simulink model "AC_SYS_SS"  (R2023b)
settings: Solver=FixedStepDiscrete  StartTime=0.0  StopTime=2  FixedStep=Ts_Power  RelTol=1e-4  EnableMultiTasking=on
PreLoadFcn:
  | HVDCMMCInterconnectionParam
StartFcn:
  | tic
StopFcn:
  | toc
values from neighbouring files (symbols this model uses):
  C_PM = 1.758e-3    (= 0.001758)    [HVDCMMCInterconnectionParam.m]
  D_R = 0.001    [HVDCMMCInterconnectionParam.m]
  D_Rs = 1e8    (= 100000000)    [HVDCMMCInterconnectionParam.m]
  Fnom = 50    [HVDCMMCInterconnectionParam.m]
  HRM = 2    [HVDCMMCInterconnectionParam.m]
  Limits_Qreg = [ 0.25, -0.25 ]    [HVDCMMCInterconnectionParam.m]
  Nb_PM = 36    [HVDCMMCInterconnectionParam.m]
  P_Ld1 = Psc/30    (= 666666666.667)    [HVDCMMCInterconnectionParam.m]
  Slope_Pref = 0.5    [HVDCMMCInterconnectionParam.m]
  Slope_Qref = 0.5    [HVDCMMCInterconnectionParam.m]
  Slope_Vdc_ref = Vnom_dc/5    (= 128000)    [HVDCMMCInterconnectionParam.m]
  Tbrk1_On = 0.1    [HVDCMMCInterconnectionParam.m]
  Tbrk2_On = 1.0    (= 1)    [HVDCMMCInterconnectionParam.m]
  Tdeblock = 1.5    [HVDCMMCInterconnectionParam.m]
  Tfault = 9999    [HVDCMMCInterconnectionParam.m]
  Ton_Converter2 = 4    [HVDCMMCInterconnectionParam.m]
  Ton_PQreg = 4    [HVDCMMCInterconnectionParam.m]
  Ton_VDCreg = 1.5    [HVDCMMCInterconnectionParam.m]
  Ts = Ts_Control    (= 4e-05)    [HVDCMMCInterconnectionParam.m]
  Ts_Power = 20e-6    (= 2e-05)    [HVDCMMCInterconnectionParam.m]
  Vb_dc = Vnom_dc    (= 640000)    [HVDCMMCInterconnectionParam.m]
  Vnom_dc = 640e3    (= 640000)    [HVDCMMCInterconnectionParam.m]
  Vnom_prim = 400e3    (= 400000)    [HVDCMMCInterconnectionParam.m]
  Vnom_sec = 333e3    (= 333000)    [HVDCMMCInterconnectionParam.m]
  w = 2*pi*Fnom    (= 314.159265359)    [HVDCMMCInterconnectionParam.m]
undefined symbols (not defined in the file or in its folder): ACSYS_T, DiscIntNeverNeededParam, Discrete, Pcc, sps_AC, spsDiodeModel
libraries: simulink x12, spsThreePhaseSeriesRLCBranchLib x7, spsGroundLib x3, spsControlledVoltageSourceLib x3, spsMultimeterLib x2, spsThreePhaseVIMeasurementLib x2, spsThreePhaseBreakerLib x1, spsThreePhaseSeriesRLCLoadLib x1, spspowerguiLib x1
(part 1 of 2)
settings Model: Creator=The MathWorks, Inc.  LastModifiedBy=rober
settings SolverCC: ConcurrentTasks=on  ZeroCrossAlgorithm=Adaptive  InsertRTBMode=Always
settings DataIOCC: SaveFormat=StructureWithTime  SaveOutput=off  SignalLogging=off  DSMLogging=off  SaveTime=off  ReturnWorkspaceOutputs=off
settings OptimizationCC: ReuseModelBlockBuffer=off  ExpressionDepthLimit=2147483647  LifeSpan=inf
settings DebuggingCC: UnderspecifiedInitializationDetection=Classic  MergeDetectMultiDrivingBlocksExec=none  SolverPrmCheckMsg=warning  FcnCallInpInsideContextMsg=warning  AllowSymbolicDim=off  StateNameClashWarn=warning  SFUnexpectedBacktrackingDiag=warning  SFNoUnconditionalDefaultTransitionDiag=warning  SFExecutionAtInitializationDiag=none  ArithmeticOperatorsInVariantConditions=warning
settings HardwareCC: ProdBitPerPointer=32  ProdBitPerSizeT=32  ProdBitPerPtrDiffT=32  ProdLargestAtomicFloat=None  ProdIntDivRoundTo=Undefined  ProdEndianess=Unspecified  ProdWordSize=32  ProdHWDeviceType=32-bit Generic
settings ModelReferenceCC: EnableRefExpFcnMdlSchedulingChecks=on  EnableParallelModelReferenceBuilds=on  ModelReferenceMinAlgLoopOccurrences=on  PropagateSignalLabelsOutOfModel=off  UseModelRefSolver=on
settings SFSimCC: SimUseLocalCustomCode=off  CustomCodeUndefinedFunction=UseInterfaceOnly
settings RTWCC: RTWUseLocalCustomCode=off
settings CodeAppCC: StateflowObjectComments=on
settings GRTTargetCC: CombineOutputUpdateFcns=off  GRTInterface=on
settings ConfigComp: CovMetricSettings=dw  CovSaveCumulativeToWorkspaceVar=on  CovSaveSingleToWorkspaceVar=on  CovExternalEMLEnable=off
settings SimscapeCC: SimscapeNormalizeSystem=off

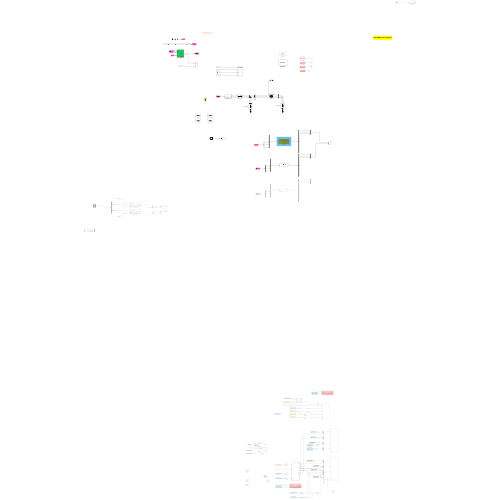
[thumbnail: Simulink's stored preview of the top-level diagram]
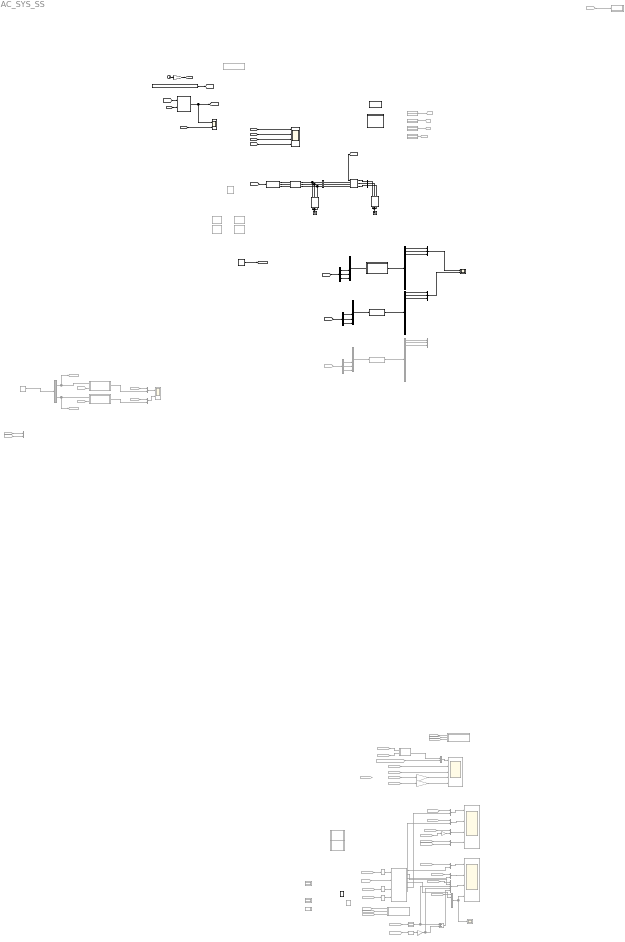
== system AC_SYS_SS ==
  note: HVDC-MMC Control System
  3ph SM1 : Subsystem  Commented=on
  3ph SM2 : Subsystem  Commented=on
  BRK_CTRL : Subsystem  Commented=on
  BRK_CTRL1 : Subsystem  Commented=on
  Brk1 : spsThreePhaseBreakerLib/Three-Phase Breaker  InitialState=open  SwitchA=on  SwitchB=on  SwitchC=on  SwitchTimes=0.1  External=on  BreakerResistance=0.0077  SnubberResistance=0.85e6  SnubberCapacitance=inf  Measurements=Breaker voltages and currents
  Brk1_RS : spsThreePhaseSeriesRLCBranchLib/Three-Phase Series RLC Branch  Commented=on  LConnTagsString=A|B|C  RConnTagsString=A|B|C  BranchType=R  Resistance=1e6  Inductance=Vnom_prim^2 / Pcc / (2*pi*Fnom)  Capacitance=1e-6  Measurements=None
  Brk1_Ron : spsThreePhaseSeriesRLCBranchLib/Three-Phase Series RLC Branch  Commented=on  LConnTagsString=A|B|C  RConnTagsString=A|B|C  BranchType=R  Resistance=0.009  Inductance=Vnom_prim^2 / Pcc / (2*pi*Fnom)  Capacitance=1e-6  Measurements=None
  Brk2_RS : spsThreePhaseSeriesRLCBranchLib/Three-Phase Series RLC Branch  Commented=on  LConnTagsString=A|B|C  RConnTagsString=A|B|C  BranchType=R  Resistance=1e6  Inductance=Vnom_prim^2 / Pcc / (2*pi*Fnom)  Capacitance=1e-6  Measurements=None
  Brk2_Ron : spsThreePhaseSeriesRLCBranchLib/Three-Phase Series RLC Branch  Commented=on  LConnTagsString=A|B|C  RConnTagsString=A|B|C  BranchType=R  Resistance=0.011  Inductance=Vnom_prim^2 / Pcc / (2*pi*Fnom)  Capacitance=1e-6  Measurements=None
  Clock : Clock
  Constant3 : Constant  Value=complex( [[ 0 Vnom_prim*sqrt(2/3); 0 0; 0 0] zeros(3,HRM-1) ])
  DQn->ABC : MATLAB Function  TreatAsAtomicUnit=on  SystemSampleTime=Ts_Power  mask{N=HRM}
      mask prompts: N "Harmonic order:"
  DSS : Subsystem  SystemSampleTime=Ts_Power  mask{A=ACSYS_T.A, B=ACSYS_T.B, C=ACSYS_T.C, D=ACSYS_T.D, InitVec=ACSYS_T.x0, dt=Ts_Power, NrBrk=3, DQSYM=off, N=HRM, Ws=w}
      mask prompts: InitVec "Initial condition:"; dt "Time step (s):"; NrBrk "Number of breakers:"; N "Harmonic number:"; Ws "Angular frequency (1/rad):"
      mask init:
      | % I = eye(size(A,1));
      | % INVR = I/(I-A*dt/2);
      | % Ad1 = INVR*(I+A*dt/2);
      | % Bd1 = INVR*B*dt/2;
      | % Cd1 = C*Ad1;
      | % Dd11 = C*INVR*B*dt/2+D;
      | % Dd12 = C*INVR*B*dt/2;
      | 
      |     I = eye(size(A,1));
      |     INVR = I/(I-A*dt/2);
      |     Ad1 = INVR*(I+A*dt/2);
      |     Bd1 = INVR*B;
      |     Cd1 = C*INVR*dt;
      |     Dd1 = Cd1*B/2 + D;
      | 
      | DQSYM = get_param(gcb,'DQSYM');
      | 
      | comp = 0;
      | 
      |     arows = size(Ad1,1)/3; %signal size
      |     acols = size(Ad1,2)/3; %signal size
      | 
      |     brows = size(Bd1,1)/3; %signal size
      |     bcols = size(Bd1,2)/3; %signal size
      | 
      |     crows = size(Cd1,1)/3; %signal size
      |     ccols = size(Cd1,2)/3; %signal size
      | 
      |     d1rows = size(Dd1,1)/3; %signal size
      |     d1cols = size(Dd1,2)/3; %signal size
      | 
      | if(strcmp(DQSYM,'on'))
      | 
      | %Calculating the PNZ matrices
      | 
      |     a = -0.5+0.866i;
      |     a2 = -0.5-0.866i;
      |     Sas = [1,a,a2;1,a2,a;1,1,1]/3;
      | 
      | 
      | 
      |     %%%%%%%%%%%%%%%%%%%%%%% Check for inconsistencies  %%%%%%%%%%%%%%%%%%%%%%%
      | 
      |     szMatA = size(A,1);
      |     iL = eye(szMatA);
      |     szMatiL = size(iL,1);
      | 
      |     if(szMatiL ~= szMatA || size(A,1) ~= size(A,2) || size(iL,1) ~= size(iL,2))
      |         error('[Int_DQN_Mat/swFeedback] check matrix A size!');
      |     end
      | 
      |     if(arows ~= brows || acols ~= ccols || crows ~= d1rows || bcols ~= d1cols)
      |         error('[Int_DQN_Mat/Initialize] the sizes of the state-space matrices!');
      |     end
      | 
      |     %%%%%%%%%%%%%%%%%%%%%%%%%%%%%%%%%%%%%%%%%%%%%%%%%%%%%%%%%%%%%%%
      | 
      | 
      |     %%%%%%%%%%%%%%%%%%%%%%% A --> Bpnz %%%%%%%%%%%%%%%%%%%%%%%
      |     Adc = complex(zeros(3*arows,3*acols));
      | 
      |     for i = 1 : arows
      |         for j = 1 : acols
      |             Adc((1:3) + (i-1)*3,(1:3) + (j-1)*3) = Sas*Ad1((1:3) + (i-1)*3,(1:3) + (j-1)*3)/Sas;
      |             %Adc((1:3) + (i-1)*3,(1:3) + (j-1)*3) = diag(diag(real(Adc((1:3) + (i-1)*3,(1:3) + (j-1)*3))));
      |             %Adc((1:3) + (i-1)*3,(1:3) + (j-1)*3) = diag(diag((Adc((1:3) + (i-1)*3,(1:3) + (j-1)*3))));
      | 
      |         end
      |     end
      |     %%%%%%%%%%%%%%%%%%%%%%%%%%%%%%%%%%%%%%%%%%%%%%%%%%%%%%%%%%%%%%%
      | 
      |     %%%%%%%%%%%%%%%%%%%%%%% B --> Bpnz %%%%%%%%%%%%%%%%%%%%%%%
      | 
      |     Bdc = complex(zeros(3*brows,3*bcols));
      | 
      |     for i = 1 : brows
      |         for j = 1 : bcols
      |             Bdc((1:3) + (i-1)*3,(1:3) + (j-1)*3) = Sas*Bd1((1:3) + (i-1)*3,(1:3) + (j-1)*3)/Sas;
      |             %Bdc((1:3) + (i-1)*3,(1:3) + (j-1)*3) = diag(diag(real(Bdc((1:3) + (i-1)*3,(1:3) + (j-1)*3))));
      |             %Bdc((1:3) + (i-1)*3,(1:3) + (j-1)*3) = diag(diag((Bdc((1:3) + (i-1)*3,(1:3) + (j-1)*3))));
      | 
      |         end
      |     end
      |     %%%%%%%%%%%%%%%%%%%%%%%%%%%%%%%%%%%%%%%%%%%%%%%%%%%%%%%%%%%%%%%
      | 
      |     %%%%%%%%%%%%%%%%%%%%%%% C --> Cpnz %%%%%%%%%%%%%%%%%%%%%%%
      | 
      |     Cdc = complex(zeros(3*crows,3*ccols));
      | 
      |     for i = 1 : crows
      |         for j = 1 : ccols
      |             Cdc((1:3) + (i-1)*3,(1:3) + (j-1)*3) = Sas*Cd1((1:3) + (i-1)*3,(1:3) + (j-1)*3)/Sas;
      |             %Cdc((1:3) + (i-1)*3,(1:3) + (j-1)*3) = diag(diag(real(Cdc((1:3) + (i-1)*3,(1:3) + (j-1)*3))));
      |             %Cdc((1:3) + (i-1)*3,(1:3) + (j-1)*3) = diag(diag((Cdc((1:3) + (i-1)*3,(1:3) + (j-1)*3))));
      |         end
      |     end
      |     %%%%%%%%%%%%%%%%%%%%%%%%%%%%%%%%%%%%%%%%%%%%%%%%%%%%%%%%%%%%%%%
      | 
      |     
      |     %%%%%%%%%%%%%%%%%%%%%%% D1 --> Cpnz %%%%%%%%%%%%%%%%%%%%%%%
      | 
      |     Ddc = complex(zeros(3*d1rows,3*d1cols));
      | 
      |     for i = 1 : d1rows
      |         for j = 1 : d1cols
      |             Ddc((1:3) + (i-1)*3,(1:3) + (j-1)*3) = Sas*Dd1((1:3) + (i-1)*3,(1:3) + (j-1)*3)/Sas;
      |             %Ddc1((1:3) + (i-1)*3,(1:3) + (j-1)*3) = diag(diag(real(Ddc1((1:3) + (i-1)*3,(1:3) + (j-1)*3))));
      |             %Ddc((1:3) + (i-1)*3,(1:3) + (j-1)*3) = diag(diag((Ddc((1:3) + (i-1)*3,(1:3) + (j-1)*3))));
      |         end
      |     end
      |     %%%%%%%%%%%%%%%%%%%%%%%%%%%%%%%%%%%%%%%%%%%%%%%%%%%%%%%%%%%%%%%
      | 
      |     Adc(abs(Adc)<2*eps) = 0;
      |     Bdc(abs(Bdc)<2*eps) = 0;
      |     Cdc(abs(Cdc)<2*eps) = 0;
      |     Ddc(abs(Ddc)<2*eps) = 0;
      | 
      |     InitVec_c = complex(zeros(brows*3,N+1));
      | 
      | 
      |     if(~isempty(InitVec))
      |         if(mod(numel(InitVec),3)~=0) 
      |             warning('[SS_DQNc_Mat] InitVec with wrong size --> needs to be a multiple of 3!'); 
      | 
      |         else
      |             for k = 1 : numel(InitVec)/3
      |                 InitVec_c((k-1)*3+1:(k-1)*3+3,1) = Sas*InitVec((k-1)*3+1:(k-1)*3+3)*exp(+1i*Ws*dt);
      |             end
      |         end
      |     end
      | 
      |     InitVec = InitVec_c;
      | 
      | 
      |     Ad1 = Adc;
      |     Bd1 = Bdc;
      |     Cd1 = Cdc;
      |     Dd1 = Ddc;
      | 
      |     comp = -1i*Ws*dt;
      | 
      | 
      | end
      | 
      |     
      |     Ad11 = Ad1(1:NrBrk,1:NrBrk);        if(isempty(Ad11)) Ad11 = zeros(3,3); end
      |     Ad12 = Ad1(1:NrBrk,NrBrk+1:end);    if(isempty(Ad12)) Ad12 = zeros(3,3); end
      |     Ad21 = Ad1(NrBrk+1:end,1:NrBrk);    if(isempty(Ad21)) Ad21 = zeros(3,3); end
      |     Ad22 = Ad1(NrBrk+1:end,NrBrk+1:end); if(isempty(Ad22)) Ad22 = zeros(3,3); end
      | 
      |     Bd11 = Bd1(1:NrBrk,1:NrBrk);        if(isempty(Bd11)) Bd11 = zeros(3,3); end
      |     Bd12 = Bd1(1:NrBrk,NrBrk+1:end);    if(isempty(Bd12)) Bd12 = zeros(3,3); end
      |     Bd21 = Bd1(NrBrk+1:end,1:NrBrk);    if(isempty(Bd21)) Bd21 = zeros(3,3); end
      |     Bd22 = Bd1(NrBrk+1:end,NrBrk+1:end); if(isempty(Bd22)) Bd22 = zeros(3,3*bcols-NrBrk); end
      | 
      |     Cd11 = Cd1(1:NrBrk,1:NrBrk);        if(isempty(Cd11)) Cd11 = zeros(3,3); end
      |     Cd12 = Cd1(1:NrBrk,NrBrk+1:end);    if(isempty(Cd12)) Cd12 = zeros(3,3); end
      |     Cd21 = Cd1(NrBrk+1:end,1:NrBrk);    if(isempty(Cd21)) Cd21 = zeros(3,3); end
      |     Cd22 = Cd1(NrBrk+1:end,NrBrk+1:end); if(isempty(Cd22)) Cd22 = zeros(3*crows-NrBrk,3*ccols); end
      | 
      |     Dd11 = Dd1(1:NrBrk,1:NrBrk);        if(isempty(Dd11)) Dd11 = zeros(3,3); end
      |     Dd12 = Dd1(1:NrBrk,NrBrk+1:end);    if(isempty(Dd12)) Dd12 = zeros(3,3); end
      |     Dd21 = Dd1(NrBrk+1:end,1:NrBrk);    if(isempty(Dd21)) Dd21 = zeros(3,3); end
      |     Dd22 = Dd1(NrBrk+1:end,NrBrk+1:end); if(isempty(Dd22)) Dd22 = zeros(3,3); end
      | 
      | 
      | 
      | 
      | InitVecS = InitVec(1:NrBrk);
      | 
      | InitVecNS = InitVec(NrBrk+1:end); if(isempty(InitVecNS)) InitVecNS = 0; end
      settings: MinAlgLoopOccurrences=on
      settings: LibrarySourceBlock=|
      | spsSynchronousMachineModel/Discrete robust/State Space Model/Discretize
      | BE or Tustin
      mask Display: disp(['{\color{red}\bf\fontsize{12}x(t) = Ad*x(t-dt)+Bd*u(t)}',newline,'{\color{gray}\bf\fontsize{12}y(t) = Cd*x(t-dt)+Dd*u(t)}'], 'texmode','on');
  Delay{,3,10..11} (4 alike) : Delay  Commented=on  DelayLength=1  SampleTime=Ts_Power
  Delay2 : Delay  DelayLength=1  SampleTime=Ts_Power
  Delay5 : Subsystem  Commented=on
  Delay6 : Subsystem  Commented=on
  Delay7 : Subsystem  Commented=on
  Delay8 : Subsystem  Commented=on
  Delay9 : Subsystem  Commented=on
  Demux : Demux  Outputs=3
  Demux1 : Demux  Outputs=3
  Demux2 : Demux  Commented=on  Outputs=3
  Demux3 : Demux  Outputs=numel(ACSYS_T.outputs)
  Demux4 : Demux  Commented=on  Outputs=2
  Demux5 : Demux  Commented=on  Outputs=numel(ACSYS_T.outputs)
  Demux6 : Demux  Outputs=numel(ACSYS_T.outputs)
  Discrete State-Space : DiscreteStateSpace  A=ACSYS_T.Adiscrete  B=ACSYS_T.Bdiscrete  C=ACSYS_T.Cdiscrete  D=ACSYS_T.Ddiscrete  InitialCondition=ACSYS_T.x0  SampleTime=Ts_Power
  Discrete State-Space1 : DiscreteStateSpace  Commented=on  A=ACSYS_T.Adiscrete  B=ACSYS_T.Bdiscrete  C=ACSYS_T.Cdiscrete  D=ACSYS_T.Ddiscrete  InitialCondition=ACSYS_T.x0  SampleTime=Ts
  From : From  Commented=on  GotoTag=Uref_Ap  TagVisibility=global
  From1 : From  Commented=on  GotoTag=Uref_An  TagVisibility=global
  From102 : From  Commented=on  GotoTag=Ap_Vin  TagVisibility=global
  From103 : From  Commented=on  GotoTag=Ap_Vbl  TagVisibility=global
  From107 : From  Commented=on  GotoTag=I_Ap_Db  TagVisibility=global
  From11 : From  Commented=on  GotoTag=Q
  From{27,44,48,113} (4 alike) : From  Commented=on  GotoTag=I_Ap_Dt  TagVisibility=global
  From118 : From  Commented=on  GotoTag=I_Ap_Db  TagVisibility=global
  From119 : From  Commented=on  GotoTag=Ap_Icap
  From{36..37,91,120} (4 alike) : From  Commented=on  GotoTag=Ap_Ipos
  From14 : From  Commented=on  GotoTag=Vsrc_ABC  TagVisibility=global
  From2 : From  Commented=on  GotoTag=P
  From25 : From  Commented=on  GotoTag=Brk1_On  TagVisibility=global
  From26 : From  Commented=on  GotoTag=UBrk1_ss
  From28 : From  Commented=on  GotoTag=U_Ap_Dt
  From29 : From  Commented=on  GotoTag=Brk2_On  TagVisibility=global
  From30 : From  Commented=on  GotoTag=IBrk2_EMT  TagVisibility=global
  From31 : From  Commented=on  GotoTag=IBrk1_EMT  TagVisibility=global
  From33 : From  Commented=on  GotoTag=UBrk2_ss
  From34 : From  Commented=on  GotoTag=Uref_Ap  TagVisibility=global
  From39 : From  Commented=on  GotoTag=U_Ap_Dt
  From4 : From  Commented=on  GotoTag=Vdc_kV
  From5 : From  Commented=on  GotoTag=V1rmsLL
  From69 : From  Commented=on  GotoTag=U_Ap_SM
  From7 : From  Commented=on  GotoTag=An_Ipos
  From85 : From  Commented=on  GotoTag=Ap_Icap
  From9 : From  Commented=on  GotoTag=An_Icap
  From90 : From  Commented=on  GotoTag=Ap_Icap
  From96 : From  Commented=on  GotoTag=Uref_Ap  TagVisibility=global
  Gain1 : Gain  Commented=on  Gain=-1
  Gain2 : Gain  Commented=on  Gain=D_Rs/(D_R+D_Rs)
  Gain4 : Gain  Commented=on  Gain=1/Vb_dc
  Gain5 : Gain  Gain=2*pi*50
  Gain7 : Gain  Commented=on  Gain=1/Vb_dc
  Goto12 : Goto  Commented=on  GotoTag=UBrk2_EMT  TagVisibility=global
  Goto13 : Goto  Commented=on  GotoTag=UBrk1_EMT  TagVisibility=global
  Ground : spsGroundLib/Ground  LConnTagsString=a
  Ground1 : spsGroundLib/Ground  LConnTagsString=a
  Ld1 : spsThreePhaseSeriesRLCLoadLib/Three-Phase Series RLC Load  Commented=on  LConnTagsString=A|B|C  Configuration=Y (grounded)  NominalVoltage=Vnom_prim  Vabc=[1e3 1e3 1e3]  Vabcp=[1e3 1e3 1e3]  NominalFrequency=Fnom  UnbalancedPower=off  ActivePower=P_Ld1  InductivePower=0  CapacitivePower=0  Pabc=[10e3 9e3 11e3]  QLabc=[100 90 110]  QCabc=[100 90 110]  Pabcp=[10e3 9e3 11e3]  QLabcp=[100 90 110]  QCabcp=[100 90 110]  Measurements=None  LoadType=constant Z
  MATLAB Function : MATLAB Function  Commented=on  TreatAsAtomicUnit=on
  MATLAB Function2 : MATLAB Function  Commented=on  SystemSampleTime=Ts_Power  mask{Ts=Ts_Power, D_R=D_R, D_Rs=D_Rs, Nb_SM=Nb_PM, C=C_PM}
      mask prompts: Ts "Time step (s):"; D_R "Resistance Ron (Ohms):"; D_Rs "Snubber resistance Rs (Ohms):"; Nb_SM "Number of submodules:"; C "Submodule capacitance (F):"
      settings: MinAlgLoopOccurrences=on
  Model1 : Subsystem  Commented=on  AncestorBlock=spsDiodeModel/Discrete  mask(DiscreteModel){}
  Model2 : Subsystem  Commented=on  AncestorBlock=spsDiodeModel/Discrete  mask(DiscreteModel){}
  Multimeter : spsMultimeterLib/Multimeter  L=6  sel=[4 5 6]  yselected={}  Gain=[1 1 1]  OutputType=Complex  PlotAtSimulationStop=off  PhasorSimulation=off
  Multimeter1 : spsMultimeterLib/Multimeter  Commented=on  L=12  sel=[1 2 3 4 5 6]  yselected={}  Gain=[1 1 1 1 1 1]  OutputType=Complex  PlotAtSimulationStop=off  PhasorSimulation=off
  Mux : Mux  Inputs=3
  Mux1 : Mux  Inputs=numel(ACSYS_T.inputs)
  Mux{8..10,13,24,28,32..35} (10 alike) : Mux  Commented=on  Inputs=2
  Mux2 : Mux  Inputs=3
  Mux23 : Mux  Inputs=numel(ACSYS_T.inputs)
  Mux29 : Mux  Commented=on  Inputs=5
  Mux3 : Mux  Commented=on  Inputs=numel(ACSYS_T.inputs)
  Mux30 : Mux  Commented=on  Inputs=5
  Mux4 : Mux  Commented=on  Inputs=3
  P (MW) : Display  Commented=on
      settings: Format=bank  Decimation=5000
  Q (Mvar) : Display  Commented=on
      settings: Format=bank  Decimation=5000
  RL Src : spsThreePhaseSeriesRLCBranchLib/Three-Phase Series RLC Branch  LConnTagsString=A|B|C  RConnTagsString=A|B|C  BranchType=RL  Resistance=0.8929  Inductance=16.58e-3  Capacitance=1e-6  Measurements=None
  R_startup1 : spsThreePhaseSeriesRLCBranchLib/Three-Phase Series RLC Branch  LConnTagsString=A|B|C  RConnTagsString=A|B|C  BranchType=R  Resistance=3200  Inductance=Vnom_prim^2 / Pcc / (2*pi*Fnom)  Capacitance=1e-6  Measurements=None
  R_startup2 : spsThreePhaseSeriesRLCBranchLib/Three-Phase Series RLC Branch  LConnTagsString=A|B|C  RConnTagsString=A|B|C  BranchType=R  Resistance=Vnom_prim^2/P_Ld1  Inductance=Vnom_prim^2 / Pcc / (2*pi*Fnom)  Capacitance=1e-6  Measurements=None
  Scope : Scope  Commented=on  NumInputPorts=2
  Scope1 : Scope  NumInputPorts=4
  Scope2 : Scope  Commented=on  NumInputPorts=5
  Scope3 : Scope  Commented=on  NumInputPorts=4
  Scope4 : Scope  NumInputPorts=2
  Scope5 : Scope  Commented=on  NumInputPorts=4
  Scope7 : Scope  Commented=on
  Scope8 : Scope  NumInputPorts=2
  Sequencer : Subsystem
      mask Display: disp('Sequencer')
  Status : From  Commented=on  GotoTag=T43_3835_2986319703090  TagVisibility=global
      settings: CloseFcn=tagdialog Close
  Status_Bottom : From  Commented=on  GotoTag=T42_3768_2839018950081  TagVisibility=global
      settings: CloseFcn=tagdialog Close
  Status_Top : From  Commented=on  GotoTag=T43_3835_2986319703090  TagVisibility=global
      settings: CloseFcn=tagdialog Close
  Subtract : Sum  Commented=on  Inputs=+-
  USW_Bottom : From  Commented=on  GotoTag=T43_3867_2942891286788  TagVisibility=global
  USW_Bottom1 : From  Commented=on  GotoTag=T43_3867_2942891286788  TagVisibility=global
  USW_Top2 : From  Commented=on  GotoTag=T44_3934_3096165412659  TagVisibility=global
  USW_Top3 : From  Commented=on  GotoTag=T44_3934_3096165412659  TagVisibility=global
  Uref2m1 : Subsystem  Commented=on
  V1 (kV rms LL) : Display  Commented=on
      settings: Format=bank  Decimation=5000
  Vdc (kV) : Display  Commented=on
      settings: Format=bank  Decimation=5000
  Voltage source : Subsystem
  param : Subsystem  Commented=on
      settings: OpenFcn=open('HVDCMMCInterconnectionParam')
      mask Display: disp('Double-click to open\nparameters file')
  powergui : spspowerguiLib/powergui  Priority=1  SimulationMode=Discrete  SampleTime=Ts_Power  frequency=60  Iterations=50  frequencyindice=0  Pbase=100e6  ErrMax=1e-4  UnitsV=kV  UnitsW=MW  buscounter=0  FunctionMessages=off  echomessages=off  EnableUseOfTLC=off  CurrentSourceSwitches=off  DisableSnubberDevices=off  DisableRonSwitches=off  DisableVfSwitches=off  DisplayEquations=off  AutomaticDiscreteSolvers=off  SolverType=Tustin/Backward Euler (TBE)  Interpol=off  ExternalGateDelay=off  methode=off  Ts=10  x0status=blocks  SPID=off  SwTol=0  HookPort=off  NonlinearTolerance=1e-4  nMaxIteration=100  ContinueOnMaxIteration=off  RestoreLinks=warning  ResistiveCurrentMeasurement=off  Frange=[0:2:500]  Ylog=off  Xlog=on  ShowGrid=off  save=off  variable=ZData  structure=VIprim  ZoomFFT=on  StartTime=0.15  cycles=2  DisplayStyle=1  fundamental=50  FreqAxis=on  MaxFrequency=1000  frequencyindicesteady=1  RmsSteady=1  display=off
  prim : spsThreePhaseVIMeasurementLib/Three-Phase V-I Measurement  VoltageMeasurement=phase-to-ground  SetLabelV=on  LabelV=Vprim  Vpu=off  VpuLL=off  CurrentMeasurement=yes  SetLabelI=on  LabelI=Iprim  Ipu=off  Pbase=100e6  Vbase=500e3  OutputType=Complex  PhasorSimulation=off  PSBequivalent=0
  sec : spsThreePhaseVIMeasurementLib/Three-Phase V-I Measurement  VoltageMeasurement=phase-to-ground  SetLabelV=on  LabelV=Vsec  Vpu=off  VpuLL=off  CurrentMeasurement=yes  SetLabelI=on  LabelI=Isec  Ipu=off  Pbase=100e6  Vbase=500e3  OutputType=Complex  PhasorSimulation=off  PSBequivalent=0
  tag scope: IBrk1_EMT=global, Vsrc_ABC=global, wt0=global
  wires:
  From2/1 -> P (MW)/1
  From4/1 -> Vdc (kV)/1
  From5/1 -> V1 (kV rms LL)/1
  From11/1 -> Q (Mvar)/1
  From/1 -> Uref2m1/1(In1)
  [Vsrc_ABC] -> Voltage source/1(In1)
  [wt0] -> DQn->ABC/2(tho)  "theta"
  [VSRC_C] -> DQn->ABC/1(Xdcpnz_c)  "[N+1,18 (6+6+6)]"
  [Vsec] -> Scope8/2
  DQn->ABC/1(Xabc) -> Scope8/1, [Vsrc_ABC]  "Mac_EMT"
  Constant3/1 -> [VSRC_C]
  Gain5/1 -> [wt0]
  Clock/1 -> Gain5/1
  From1/1 -> 3ph SM1/1(Uref_An)
  From7/1 -> 3ph SM1/2(An_Ipos)
  From9/1 -> 3ph SM1/3(An_Icap)
  From27/1 -> Scope2/2  "U_Ap_Dt"
  From28/1 -> Scope2/3  "U_Ap_Dt"
  From102/1 -> Gain4/1  "Ap_Vin"
  From103/1 -> Gain7/1  "Ap_Vbl"
  Status/1 -> Mux9/2  "Status"
  Gain4/1 -> Scope2/4  "Ap_Vin"
  Gain7/1 -> Scope2/5  "Ap_Vbl"
  Mux9/1 -> Scope2/1
  MATLAB Function/2(status) -> Mux9/1
  From44/1 -> MATLAB Function/1(Id)  "U_Ap_Dt"
  From39/1 -> MATLAB Function/2(Vd)  "U_Ap_Dt"
  ? -> Model2/1(Uswitch)  "USW_Bottom_fcn"
  ? -> Model2/2(status)  "Status_Bottom_Fcn"
  ? -> Model1/1(Uswitch)  "USW_Top"
  ? -> Model1/2(status)  "Status_Top"
  From85/1 -> 3ph SM2/3(Ap_Icap)
  From34/1 -> 3ph SM2/1(Uref_Ap)
  From36/1 -> 3ph SM2/2(Ap_Ipos)
  From91/1 -> Delay10/1  "Ap_Icap"
  From69/1 -> Delay3/1  "U_Ap_SM"
  From90/1 -> Delay11/1  "Ap_Ipos"
  Delay11/1 -> MATLAB Function2/4(Ic)
  Delay10/1 -> MATLAB Function2/3(Ip)
  Delay3/1 -> MATLAB Function2/1(Usm)
  MATLAB Function2/1(UDt) -> Mux24/2  "USW_Top_fcn"
  USW_Top2/1 -> Mux24/1  "USW_Top"
  Mux24/1 -> Scope3/1
  Mux28/1 -> Scope3/2
  USW_Bottom/1 -> Mux28/1  "USW_Bottom"
  MATLAB Function2/3(UDb) -> Mux28/2  "USW_Bottom_fcn"
  Mux29/1 -> Scope3/3
  Status_Top/1 -> Mux29/1  "Status_Top"
  MATLAB Function2/2(Stt) -> Mux29/2  "Status_Top"
  Mux30/1 -> Scope3/4, Scope7/1
  Status_Bottom/1 -> Mux30/1  "Status_Bottom"
  MATLAB Function2/4(Stb) -> Mux30/2  "Status_Bottom_Fcn"
  Mux35/1 -> Scope5/4
  Mux33/1 -> Scope5/2
  Mux34/1 -> Scope5/3
  Mux32/1 -> Scope5/1
  From118/1 -> Mux35/2
  MATLAB Function2/6(IDb) -> Mux33/2  "Db_fcn"
  MATLAB Function2/5(IDt) -> Mux32/2  "Dt_fcn"
  From48/1 -> Mux32/1  "I_Ap_Dt"
  From107/1 -> Mux33/1  "I_Ap_Db"
  USW_Top3/1 -> Mux34/1  "USW_Top"
  Gain1/1 -> Mux34/2
  USW_Bottom1/1 -> Gain1/1  "USW_Bottom"
  From113/1 -> Mux35/1  "I_Ap_Dt"
  From119/1 -> Delay8/1(In1)  "Ap_Ipos"
  Delay9/1(Out1) -> Mux29/3, Subtract/1  "Ipos"
  From120/1 -> Delay9/1(In1)  "Ap_Icap"
  Delay8/1(Out1) -> Gain2/1  "Icap"
  Gain2/1 -> Mux29/4, Subtract/2
  Subtract/1 -> Mux29/5  "Ib"
  From96/1 -> MATLAB Function2/2(Uref)
  DSS/1(Y) -> Demux6/1
  Mux23/1 -> DSS/1(U)
  From26/1 -> Mux13/1  "UBrk1_EMT"
  From33/1 -> Mux13/2  "UBrk2_EMT"
  Multimeter1/1 -> Demux4/1
  Demux4/1 -> Goto13/1, BRK_CTRL/1(UBrk1_EMT)  "UBrk1_EMT"
  From25/1 -> BRK_CTRL/2(Brk_ON)
  From29/1 -> BRK_CTRL1/2(Brk_ON)
  Demux4/2 -> Goto12/1, BRK_CTRL1/1(UBrk1_EMT)  "UBrk2_EMT"
  Mux8/1 -> Scope/1
  Mux10/1 -> Scope/2
  From31/1 -> Mux8/1
  From30/1 -> Mux10/1
  BRK_CTRL/1(IBrk1_ss) -> Mux8/2  "IBrk1_ss"
  BRK_CTRL1/1(IBrk1_ss) -> Mux10/2  "IBrk2_ss"
  [Brk1_On] -> Brk1/1
  [Vsec] -> Scope1/2
  [Vprim] -> Scope1/1
  [Isec] -> Scope1/4
  [Iprim] -> Scope1/3
  Multimeter/1 -> [IBrk1_EMT]
  Demux/1 -> Mux23/4
  Demux/2 -> Mux23/5
  Demux/3 -> Mux23/6
  [Vsrc_ABC] -> Demux/1
  Demux1/3 -> Mux1/6
  [Vsrc_ABC] -> Demux1/1
  Demux1/2 -> Mux1/5
  Mux1/1 -> Discrete State-Space/1
  Demux1/1 -> Mux1/4
  Discrete State-Space/1 -> Demux3/1
  Demux6/1 -> Mux/1
  Demux6/2 -> Mux/2
  Demux6/3 -> Mux/3
  Demux3/1 -> Mux2/1
  Demux3/3 -> Mux2/3
  Demux3/2 -> Mux2/2
  Mux3/1 -> Discrete State-Space1/1
  From14/1 -> Demux2/1
  Discrete State-Space1/1 -> Demux5/1
  Demux5/2 -> Mux4/2
  Demux2/1 -> Mux3/4
  Demux2/2 -> Mux3/5
  Demux5/1 -> Mux4/1
  Demux5/3 -> Mux4/3
  Demux2/3 -> Mux3/6
  Mux/1 -> Scope4/1
  Mux2/1 -> Scope4/2
  connections:
  RL Src/RConn1 -- prim/RConn1 -- R_startup2/LConn1
  RL Src/RConn2 -- prim/RConn2 -- R_startup2/LConn2
  RL Src/RConn3 -- prim/RConn3 -- R_startup2/LConn3
  Voltage source/RConn3 -- RL Src/LConn3
  Voltage source/RConn2 -- RL Src/LConn2
  Voltage source/RConn1 -- RL Src/LConn1
  Brk1/LConn1 -- prim/LConn1
  Brk1/LConn2 -- prim/LConn2
  Brk1/LConn3 -- prim/LConn3
  R_startup1/LConn1 -- sec/LConn1
  R_startup1/LConn2 -- sec/LConn2
  R_startup1/LConn3 -- sec/LConn3
  Ground/LConn1 -- R_startup1/RConn3 -- R_startup1/RConn1 -- R_startup1/RConn2
  Ground1/LConn1 -- R_startup2/RConn3 -- R_startup2/RConn1 -- R_startup2/RConn2
  Brk1/RConn3 -- sec/RConn3
  Brk1/RConn2 -- sec/RConn2
  Brk1/RConn1 -- sec/RConn1

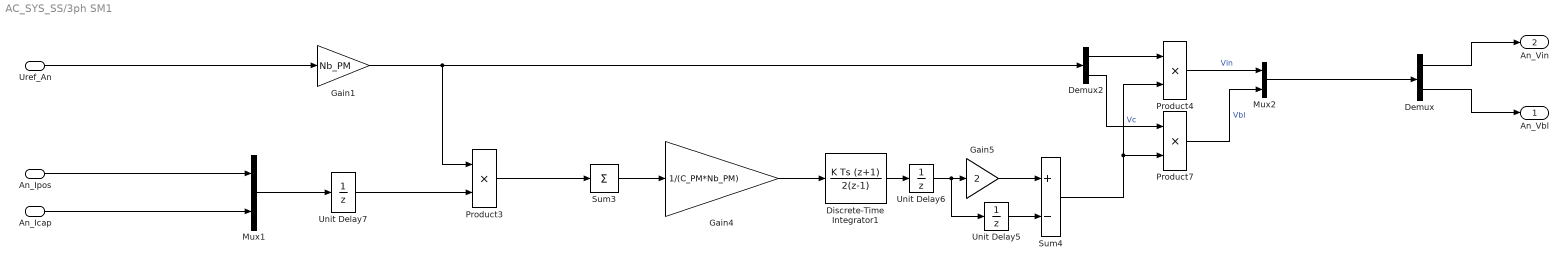
== system AC_SYS_SS/3ph SM1 ==
  Uref_An : Inport
  An_Ipos : Inport  Port=2
  An_Icap : Inport  Port=3
  Demux : Demux  Outputs=2
  Demux2 : Demux  Outputs=2
  Discrete-Time Integrator1 : DiscreteIntegrator  IntegratorMethod=Integration: Trapezoidal  gainval=1  SampleTime=Ts_Power  UpperSaturationLimit=5000  LowerSaturationLimit=500  ICPrevOutput=DiscIntNeverNeededParam  ICPrevScaledInput=DiscIntNeverNeededParam
  Gain1 : Gain  Gain=Nb_PM
  Gain4 : Gain  Gain=1/(C_PM*Nb_PM)
  Gain5 : Gain  Gain=2
  Mux1 : Mux  Inputs=2
  Mux2 : Mux  Inputs=2
  Product3 : Product
  Product4 : Product
  Product7 : Product
  Sum3 : Sum  Inputs=1  InputSameDT=on  SaturateOnIntegerOverflow=on  OutDataTypeStr=Inherit: Same as first input
  Sum4 : Sum  Inputs=+-  InputSameDT=on  SaturateOnIntegerOverflow=on  OutDataTypeStr=Inherit: Same as first input
  Unit Delay5 : UnitDelay  SampleTime=Ts_Power  HasFrameUpgradeWarning=on
  Unit Delay6 : UnitDelay  SampleTime=Ts_Power  HasFrameUpgradeWarning=on
  Unit Delay7 : UnitDelay  SampleTime=Ts_Power  HasFrameUpgradeWarning=on
  An_Vbl : Outport
  An_Vin : Outport  Port=2
  wires:
  Gain5/1 -> Sum4/1
  Gain1/1 -> Demux2/1, Product3/1
  Mux2/1 -> Demux/1
  Demux/1 -> An_Vin/1
  Uref_An/1 -> Gain1/1
  Gain4/1 -> Discrete-Time Integrator1/1
  Mux1/1 -> Unit Delay7/1
  Demux2/2 -> Product7/1
  Unit Delay6/1 -> Gain5/1, Unit Delay5/1
  An_Icap/1 -> Mux1/2
  Demux2/1 -> Product4/1
  Discrete-Time Integrator1/1 -> Unit Delay6/1
  Sum4/1 -> Product7/2, Product4/2  "Vc"
  Unit Delay5/1 -> Sum4/2
  Sum3/1 -> Gain4/1
  Product3/1 -> Sum3/1
  Product4/1 -> Mux2/1  "Vin"
  Demux/2 -> An_Vbl/1
  Product7/1 -> Mux2/2  "Vbl"
  Unit Delay7/1 -> Product3/2
  An_Ipos/1 -> Mux1/1

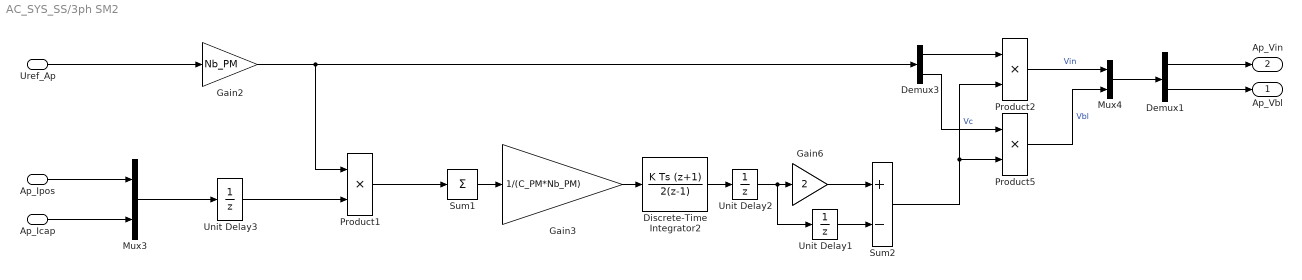
== system AC_SYS_SS/3ph SM2 ==
  Uref_Ap : Inport
  Ap_Ipos : Inport  Port=2
  Ap_Icap : Inport  Port=3
  Demux1 : Demux  Outputs=2
  Demux3 : Demux  Outputs=2
  Discrete-Time Integrator2 : DiscreteIntegrator  IntegratorMethod=Integration: Trapezoidal  gainval=1  SampleTime=Ts_Power  UpperSaturationLimit=5000  LowerSaturationLimit=500  ICPrevOutput=DiscIntNeverNeededParam  ICPrevScaledInput=DiscIntNeverNeededParam
  Gain2 : Gain  Gain=Nb_PM
  Gain3 : Gain  Gain=1/(C_PM*Nb_PM)
  Gain6 : Gain  Gain=2
  Mux3 : Mux  Inputs=2
  Mux4 : Mux  Inputs=2
  Product1 : Product
  Product2 : Product
  Product5 : Product
  Sum1 : Sum  Inputs=1  InputSameDT=on  SaturateOnIntegerOverflow=on  OutDataTypeStr=Inherit: Same as first input
  Sum2 : Sum  Inputs=+-  InputSameDT=on  SaturateOnIntegerOverflow=on  OutDataTypeStr=Inherit: Same as first input
  Unit Delay1 : UnitDelay  SampleTime=Ts_Power  HasFrameUpgradeWarning=on
  Unit Delay2 : UnitDelay  SampleTime=Ts_Power  HasFrameUpgradeWarning=on
  Unit Delay3 : UnitDelay  SampleTime=Ts_Power  HasFrameUpgradeWarning=on
  Ap_Vbl : Outport
  Ap_Vin : Outport  Port=2
  wires:
  Demux1/2 -> Ap_Vbl/1
  Ap_Ipos/1 -> Mux3/1
  Unit Delay3/1 -> Product1/2
  Product1/1 -> Sum1/1
  Sum1/1 -> Gain3/1
  Unit Delay1/1 -> Sum2/2
  Sum2/1 -> Product5/2, Product2/2  "Vc"
  Uref_Ap/1 -> Gain2/1
  Unit Delay2/1 -> Gain6/1, Unit Delay1/1
  Mux3/1 -> Unit Delay3/1
  Demux3/2 -> Product5/1
  Gain3/1 -> Discrete-Time Integrator2/1
  Gain2/1 -> Demux3/1, Product1/1
  Demux3/1 -> Product2/1
  Demux1/1 -> Ap_Vin/1
  Mux4/1 -> Demux1/1
  Product2/1 -> Mux4/1  "Vin"
  Discrete-Time Integrator2/1 -> Unit Delay2/1
  Ap_Icap/1 -> Mux3/2
  Gain6/1 -> Sum2/1
  Product5/1 -> Mux4/2  "Vbl"

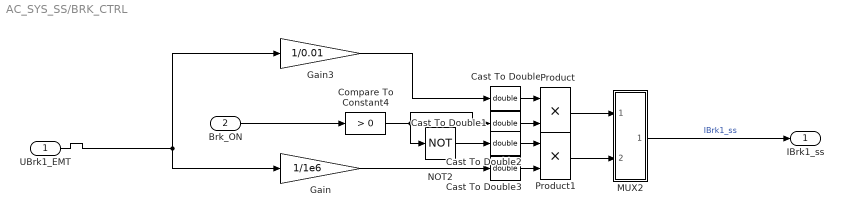
== system AC_SYS_SS/BRK_CTRL ==
  UBrk1_EMT : Inport
  Brk_ON : Inport  Port=2
  Cast To Double{,1..3} (4 alike) : DataTypeConversion  OutDataTypeStr=double  SaturateOnIntegerOverflow=off  RndMeth=Floor
  Compare To Constant4 : simulink/Logic and Bit Operations/Compare To Constant  relop=>  const=0  OutDataTypeStr=boolean
  Gain : Gain  Gain=1/1e6
  Gain3 : Gain  Gain=1/0.01
  MUX2 : Subsystem
  NOT2 : Logic  Operator=NOT  IconShape=distinctive  AllPortsSameDT=off  OutDataTypeStr=boolean
  Product : Product
  Product1 : Product
  IBrk1_ss : Outport
  wires:
  Cast To Double1/1 -> Product/2
  Product1/1 -> MUX2/2(In2)
  UBrk1_EMT/1 -> Gain3/1, Gain/1
  Compare To Constant4/1 -> Cast To Double1/1, NOT2/1
  Product/1 -> MUX2/1(In1)
  Gain/1 -> Cast To Double3/1
  NOT2/1 -> Cast To Double2/1
  Cast To Double/1 -> Product/1
  Gain3/1 -> Cast To Double/1
  Cast To Double3/1 -> Product1/2
  Brk_ON/1 -> Compare To Constant4/1
  Cast To Double2/1 -> Product1/1
  MUX2/1(Out1) -> IBrk1_ss/1  "IBrk1_ss"

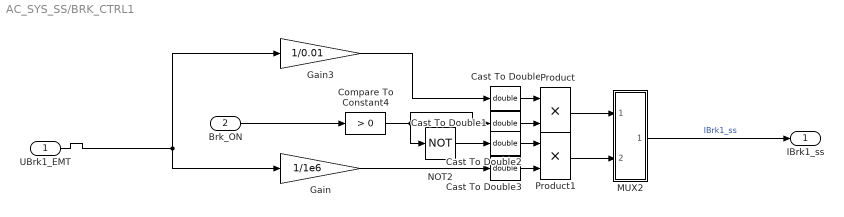
== system AC_SYS_SS/BRK_CTRL1 ==
  UBrk1_EMT : Inport
  Brk_ON : Inport  Port=2
  Cast To Double{,1..3} (4 alike) : DataTypeConversion  OutDataTypeStr=double  SaturateOnIntegerOverflow=off  RndMeth=Floor
  Compare To Constant4 : simulink/Logic and Bit Operations/Compare To Constant  relop=>  const=0  OutDataTypeStr=boolean
  Gain : Gain  Gain=1/1e6
  Gain3 : Gain  Gain=1/0.01
  MUX2 : Subsystem
  NOT2 : Logic  Operator=NOT  IconShape=distinctive  AllPortsSameDT=off  OutDataTypeStr=boolean
  Product : Product
  Product1 : Product
  IBrk1_ss : Outport
  wires:
  Cast To Double1/1 -> Product/2
  Product1/1 -> MUX2/2(In2)
  UBrk1_EMT/1 -> Gain3/1, Gain/1
  Compare To Constant4/1 -> Cast To Double1/1, NOT2/1
  Product/1 -> MUX2/1(In1)
  Gain/1 -> Cast To Double3/1
  NOT2/1 -> Cast To Double2/1
  Cast To Double/1 -> Product/1
  Gain3/1 -> Cast To Double/1
  Cast To Double3/1 -> Product1/2
  Brk_ON/1 -> Compare To Constant4/1
  Cast To Double2/1 -> Product1/1
  MUX2/1(Out1) -> IBrk1_ss/1  "IBrk1_ss"

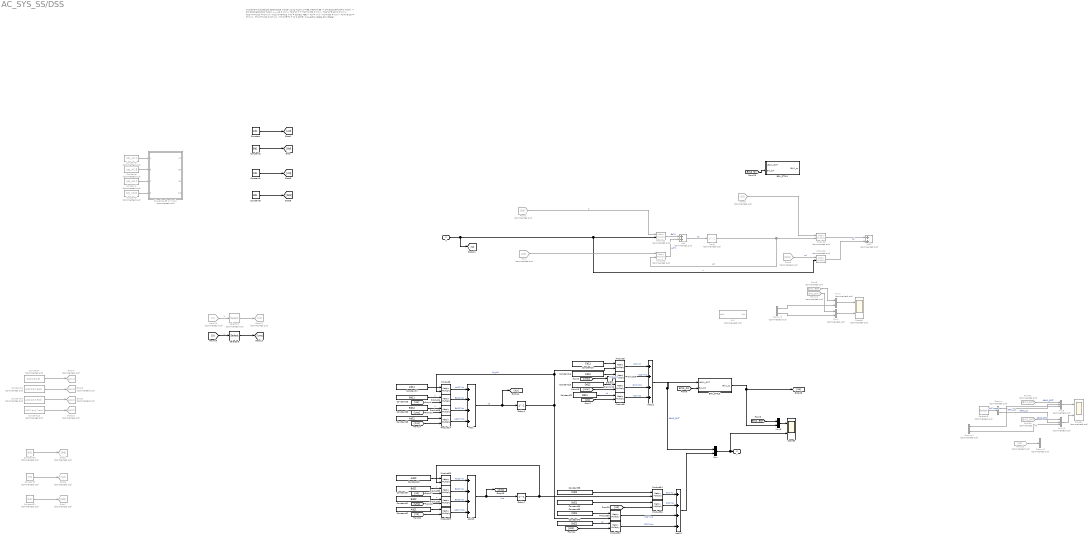
== system AC_SYS_SS/DSS ==
  note: Implement discretized state-space model using Tustin or TBE method
      |
      | BE      -> SM.DSSmethod=1
      | Tustin  -> SM.DSSmethod=2
      |
      |
      | Tustin
      | ------
      | Ad = inv(I - Ts/2*A)*(I + Ts/2*A)
      | Bd = inv(I - Ts/2*A)*B
      | Cd = C*inv(I - Ts/2*A)*Ts
      | Dd = C*inv(I - Ts/2*A)*B*Ts/2  + D  =  Cd*B/2
      |
      | TBE
      | ---
      | Ad = inv(I - Ts*A)
      | Bd = inv(I - Ts*A)*B
      | Cd = C*inv(I - Ts*A)*Ts
      | Dd = C*inv(I - Ts*A)*B*Ts  + D  =  Cd*B
      |
      | I = eye(SM.nState,SM.nState)
  U : Inport
  Add : Sum  Commented=on
  Add{1,10..12} (4 alike) : Sum  Inputs=++++
  Add2 : Sum  Commented=on
  BRK_CTRL1 : Subsystem
  BRK_CTRL3 : Subsystem
  Constant : Constant  Value=Ad1
  Constant1 : Constant  Value=Cd1
  Constant10 : Constant  Commented=on  Value=Bd1
  Constant11 : Constant  Commented=on  Value=Dd1
  Constant12 : Constant  Commented=on  Value=Ad1(1:6,7:end)
  Constant13 : Constant  Commented=on  Value=Ad1(7:end,7:end)
  Constant14 : Constant  Commented=on  Value=Ad1(1:6,7:end)
  Constant15 : Constant  Value=Ad12
  Constant16 : Constant  Value=Cd12
  Constant17 : Constant  Value=Ad11
  Constant18 : Constant  Value=Bd11
  Constant19 : Constant  Value=Cd11
  Constant2 : Constant  Value=Bd1
  Constant21 : Constant  Value=Dd11
  Constant23 : Constant  Value=Dd12
  Constant28 : Constant  Value=Bd12
  Constant3 : Constant  Value=Dd1
  Constant35 : Constant  Value=Cd21
  Constant37 : Constant  Value=Bd21
  Constant38 : Constant  Value=Cd22
  Constant39 : Constant  Value=Dd21
  Constant4 : Constant  Commented=on  Value=Ad1(1:6,1:6)
  Constant40 : Constant  Value=Dd22
  Constant41 : Constant  Value=Bd22
  Constant42 : Constant  Value=Ad21
  Constant43 : Constant  Value=Ad22
  Constant5 : Constant  Commented=on  Value=sps_AC.A
  Constant6 : Constant  Commented=on  Value=sps_AC.B
  Constant7 : Constant  Commented=on  Value=sps_AC.C
  Constant8 : Constant  Commented=on  Value=sps_AC.D
  Constant9 : Constant  Commented=on  Value=Cd1
  Delay : Delay  Commented=on  DelayLength=1  InitialCondition=InitVec  SampleTime=dt
  Delay1 : Delay  DelayLength=1  InitialCondition=InitVecS  SampleTime=dt
  Delay2 : Delay  DelayLength=1  InitialCondition=InitVecNS  SampleTime=dt
  Delay7 : Delay  DelayLength=1  InitialCondition=InitVecNS  SampleTime=dt
  Demux{,1..3} (4 alike) : Demux  Commented=on  Outputs=2
  Discretize BE or Tustin : Subsystem  Commented=on  AncestorBlock="DQN_Machines/DQN_Mac_V1/Discretize  BE or Tustin"
  From : From  Commented=on  GotoTag=Ad
  From1 : From  Commented=on  GotoTag=Bd
  From10 : From  Commented=on  GotoTag=IBrk2_EMT  TagVisibility=global
  From15 : From  Commented=on  GotoTag=U
  From2 : From  Commented=on  GotoTag=Cd
  From23 : From  Commented=on  GotoTag=Us
  From3 : From  Commented=on  GotoTag=Dd1
  From30 : From  Commented=on  GotoTag=UBrk2_EMT  TagVisibility=global
  From31 : From  Commented=on  GotoTag=UBrk1_EMT  TagVisibility=global
  From8 : From  Commented=on  GotoTag=IBrk1_EMT  TagVisibility=global
  Goto10 : Goto  Commented=on  GotoTag=Ad22
  Goto12 : Goto  Commented=on  GotoTag=Us
  Goto2 : Goto  Commented=on  GotoTag=Bd
  Goto4 : Goto  Commented=on  GotoTag=Ad11
  Goto6 : Goto  Commented=on  GotoTag=Cd
  Goto7 : Goto  Commented=on  GotoTag=Dd1
  Goto8 : Goto  Commented=on  GotoTag=Ad12
  Goto9 : Goto  Commented=on  GotoTag=Ad21
  Mux : Mux  Inputs=2
  Mux1 : Mux  Commented=on  Inputs=2
  Mux10 : Mux  Commented=on  Inputs=3
  Mux2 : Mux  Commented=on  Inputs=2
  Mux3 : Mux  Inputs=2
  Mux8 : Mux  Commented=on  Inputs=3
  Product{1..2,5,7} (4 alike) : Product  Commented=on  Multiplication=Matrix(*)  SaturateOnIntegerOverflow=on  OutDataTypeStr=Inherit: Same as first input
  Product{3..4,6,8,14..15,20,28..36} (16 alike) : Product  Multiplication=Matrix(*)  SaturateOnIntegerOverflow=on  OutDataTypeStr=Inherit: Same as first input
  Scope1 : Scope  Commented=on  NumInputPorts=2
  Scope2 : Scope  Commented=on  NumInputPorts=2
  Scope3 : Scope  NumInputPorts=2
  Selector2 : Selector  Commented=on  InputPortWidth=size(B,2)  IndexOptions=Index vector (dialog)  Indices=[1:NrBrk]  OutputSizes=1
  Selector3 : Selector  Commented=on  InputPortWidth=33  IndexOptions=Index vector (dialog)  Indices=[1:6]  OutputSizes=1
  Selector6 : Selector  InputPortWidth=size(B,2)  IndexOptions=Index vector (dialog)  Indices=[NrBrk+1:size(B,2)]  OutputSizes=1
  U-I2 : Subsystem  Commented=on
  Y : Outport
  wires:
  Constant/1 -> [Ad]
  Constant2/1 -> [Bd]
  Constant1/1 -> [Cd]
  Constant3/1 -> [Dd1]
  Constant7/1 -> Discretize BE or Tustin/3(C)
  Constant6/1 -> Discretize BE or Tustin/2(B)
  Constant8/1 -> Discretize BE or Tustin/4(D)
  Constant5/1 -> Discretize BE or Tustin/1(A)
  Product2/1 -> Add2/1
  U/1 -> [U], Product7/2, Product1/2  "u"
  From1/1 -> Product1/1  "u"
  Delay/1 -> Product2/2, Product5/2  "xd"
  From3/1 -> Product7/1  "xd"
  Product1/1 -> Add/1  "Bd*U"
  Product7/1 -> Add2/2  "xd"
  Product5/1 -> Add/2  "Ad*X"
  From2/1 -> Product2/1
  From/1 -> Product5/1
  [Brk2_On] -> BRK_CTRL1/2(Brk_ON)
  ? -> BRK_CTRL1/1(UBrk1_EMT)  "UBrk2_EMT"
  Demux/2 -> Mux10/2  "IBrk2_ss"
  Mux10/1 -> Scope1/2
  From31/1 -> Mux8/1  "UBrk1_EMT"
  Mux8/1 -> Scope1/1
  From30/1 -> Mux10/1  "UBrk2_EMT"
  Demux/1 -> Mux8/2  "IBrk1_ss"
  Selector3/1 -> Demux/1  "Cd*Xnew"
  Constant4/1 -> Goto4/1
  Constant10/1 -> Goto2/1
  Constant9/1 -> Goto6/1
  Constant11/1 -> Goto7/1
  Constant12/1 -> Goto8/1
  Constant14/1 -> Goto9/1
  Constant13/1 -> Goto10/1
  Constant19/1 -> Product6/1
  Delay1/1 -> Product6/2, Product8/2, Product30/2  "Xs_old"
  Add1/1 -> [Xs], Delay1/1  "Xs"
  Constant18/1 -> Product4/1  "u"
  Constant17/1 -> Product8/1
  [Us] -> Product4/2
  From15/1 -> Selector2/1  "u"
  Selector2/1 -> Goto12/1
  [U] -> Selector6/1  "u"
  Selector6/1 -> [Uns]
  Demux1/1 -> Mux8/3
  Demux1/2 -> Mux10/3
  Constant15/1 -> Product14/1
  Product14/1 -> Add1/4  "Ad12*Xns"
  Constant16/1 -> Product15/1
  [Uns] -> Product20/2
  Constant23/1 -> Product20/1  "xd"
  Add/1 -> Delay/1  "xd"
  Delay7/1 -> Product34/2, Product35/2
  [Xns] -> Product14/2
  Product8/1 -> Add1/1  "Ad11*Xs"
  Product4/1 -> Add1/2  "Bd11*Us"
  Product28/1 -> Add1/3  "Bd12*Us"
  Constant28/1 -> Product28/1  "u"
  [Uns] -> Product28/2
  Product31/1 -> Add11/4  "D12*Uns"
  Product35/1 -> Add10/1  "Ad22*Xs"
  Constant40/1 -> Product31/1  "xd"
  Product30/1 -> Add11/3  "C12*Xns"
  Product32/1 -> Add10/3  "Bd22*Us"
  Product36/1 -> Add11/2  "D11*Us"
  Constant41/1 -> Product32/1  "u"
  Constant38/1 -> Product34/1
  Constant42/1 -> Product29/1
  Product34/1 -> Add11/1  "C11*Xs"
  Product33/1 -> Add10/2  "Bd21*Us"
  Constant43/1 -> Product35/1
  Constant37/1 -> Product33/1  "u"
  [Xs] -> Product29/2
  [Uns] -> Product32/2
  [Uns] -> Product31/2
  [Us] -> Product33/2
  Add10/1 -> [Xns], Delay7/1  "Xns"
  Constant35/1 -> Product30/1
  Constant39/1 -> Product36/1
  Product29/1 -> Add10/4  "Ad21*Xns"
  From23/1 -> Demux2/1
  Product15/1 -> Add12/2  "C12*Xns"
  Product20/1 -> Add12/3  "D12*Uns"
  From10/1 -> Mux2/1
  Mux2/1 -> Scope2/2
  Mux1/1 -> Scope2/1
  From8/1 -> Mux1/1
  ? -> Demux3/1
  Demux3/2 -> Mux2/2
  Demux3/1 -> Mux1/2
  Add11/1 -> Mux/2
  Mux/1 -> Scope3/2, Y/1
  Product6/1 -> Add12/1  "C11*Xs"
  [Xns] -> Delay2/1
  Delay2/1 -> Product15/2  "Xns_old"
  Constant21/1 -> Product3/1  "xd"
  [Brk1_On] -> BRK_CTRL3/2(Brk_ON)
  [Us] -> Product3/2
  BRK_CTRL3/1(IBrk1_ss) -> Mux3/2, [Us]
  [Us] -> Product36/2
  Mux3/1 -> Scope3/1
  [IBrk1_EMT] -> Mux3/1
  Add12/1 -> Mux/1, BRK_CTRL3/1(UBrk1_EMT)  "UBrk1_EMT"
  Product3/1 -> Add12/4  "D11*Us"

== system AC_SYS_SS/Delay5 ==
  In1 : Inport
  Gain3 : Gain  Gain=0.5
  Sum4 : Sum  InputSameDT=on  SaturateOnIntegerOverflow=on  OutDataTypeStr=Inherit: Same as first input
  Unit Delay6 : UnitDelay  SampleTime=Ts_Power  HasFrameUpgradeWarning=on
  Out1 : Outport
  wires:
  In1/1 -> Sum4/2, Unit Delay6/1
  Unit Delay6/1 -> Sum4/1
  Sum4/1 -> Gain3/1
  Gain3/1 -> Out1/1

== system AC_SYS_SS/Delay6 ==
  In1 : Inport
  Gain3 : Gain  Gain=0.5
  Sum4 : Sum  InputSameDT=on  SaturateOnIntegerOverflow=on  OutDataTypeStr=Inherit: Same as first input
  Unit Delay6 : UnitDelay  SampleTime=Ts_Power  HasFrameUpgradeWarning=on
  Out1 : Outport
  wires:
  In1/1 -> Sum4/2, Unit Delay6/1
  Unit Delay6/1 -> Sum4/1
  Sum4/1 -> Gain3/1
  Gain3/1 -> Out1/1

== system AC_SYS_SS/Delay7 ==
  In1 : Inport
  Gain3 : Gain  Gain=0.5
  Sum4 : Sum  InputSameDT=on  SaturateOnIntegerOverflow=on  OutDataTypeStr=Inherit: Same as first input
  Unit Delay6 : UnitDelay  SampleTime=Ts_Power  HasFrameUpgradeWarning=on
  Out1 : Outport
  wires:
  In1/1 -> Sum4/2, Unit Delay6/1
  Unit Delay6/1 -> Sum4/1
  Sum4/1 -> Gain3/1
  Gain3/1 -> Out1/1

== system AC_SYS_SS/Delay8 ==
  In1 : Inport
  Gain3 : Gain  Gain=0.5
  Sum4 : Sum  InputSameDT=on  SaturateOnIntegerOverflow=on  OutDataTypeStr=Inherit: Same as first input
  Unit Delay6 : UnitDelay  SampleTime=Ts_Power  HasFrameUpgradeWarning=on
  Out1 : Outport
  wires:
  In1/1 -> Sum4/2, Unit Delay6/1
  Unit Delay6/1 -> Sum4/1
  Sum4/1 -> Gain3/1
  Gain3/1 -> Out1/1

== system AC_SYS_SS/Delay9 ==
  In1 : Inport
  Gain3 : Gain  Gain=0.5
  Sum4 : Sum  InputSameDT=on  SaturateOnIntegerOverflow=on  OutDataTypeStr=Inherit: Same as first input
  Unit Delay6 : UnitDelay  SampleTime=Ts_Power  HasFrameUpgradeWarning=on
  Out1 : Outport
  wires:
  In1/1 -> Sum4/2, Unit Delay6/1
  Unit Delay6/1 -> Sum4/1
  Sum4/1 -> Gain3/1
  Gain3/1 -> Out1/1

== system AC_SYS_SS/Model1 ==
  Uswitch : Inport
  status : Inport  Port=2
  0 1 : Constant  Value=0
  Gain : Gain  Gain=1./D_R  SaturateOnIntegerOverflow=on  OutDataTypeStr=Inherit: Same as input  ParamDataTypeStr=Inherit: Same as input
  Saturation : Saturate  UpperLimit=inf  LowerLimit=0
  Switch : Switch  Threshold=0.5  SaturateOnIntegerOverflow=off
  iSwitch : Outport
  wires:
  Uswitch/1 -> Gain/1
  Gain/1 -> Switch/1
  0 1/1 -> Switch/3
  Switch/1 -> Saturation/1
  Saturation/1 -> iSwitch/1
  status/1 -> Switch/2

== system AC_SYS_SS/Model2 ==
  Uswitch : Inport
  status : Inport  Port=2
  0 1 : Constant  Value=0
  Gain : Gain  Gain=1./D_R  SaturateOnIntegerOverflow=on  OutDataTypeStr=Inherit: Same as input  ParamDataTypeStr=Inherit: Same as input
  Saturation : Saturate  UpperLimit=inf  LowerLimit=0
  Switch : Switch  Threshold=0.5  SaturateOnIntegerOverflow=off
  iSwitch : Outport
  wires:
  Uswitch/1 -> Gain/1
  Gain/1 -> Switch/1
  0 1/1 -> Switch/3
  Switch/1 -> Saturation/1
  Saturation/1 -> iSwitch/1
  status/1 -> Switch/2

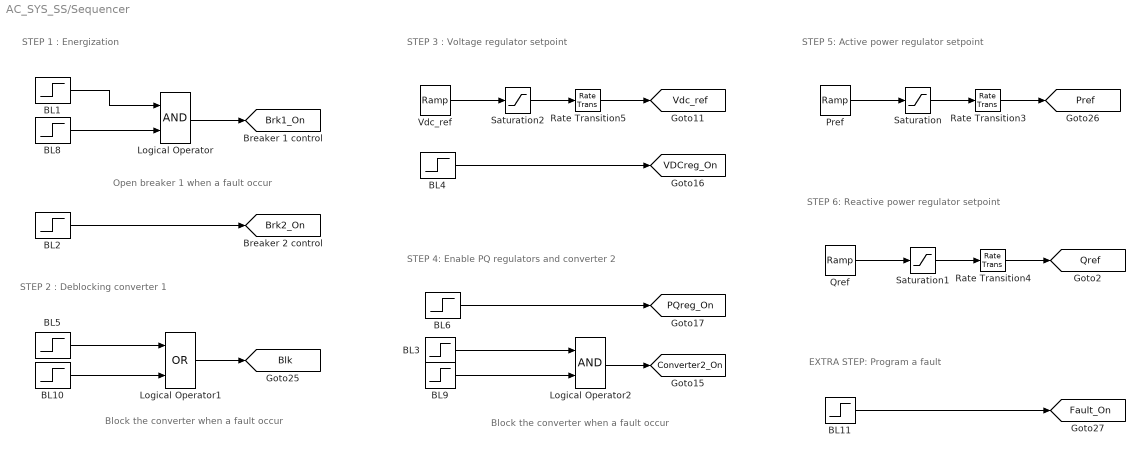
== system AC_SYS_SS/Sequencer ==
  note: Open breaker 1 when a fault occur
  note: Block the converter when a fault occur
  note: Block the converter when a fault occur
  note: STEP 6: Reactive power regulator setpoint
  note: STEP 4: Enable PQ regulators and converter 2
  note: STEP 5: Active power regulator setpoint
  note: STEP 3 : Voltage regulator setpoint
  note: STEP 2 : Deblocking converter 1
  note: STEP 1 : Energization
  note: EXTRA STEP: Program a fault
  BL1 : Step  Time=Tbrk1_On  SampleTime=Ts_Power
  BL10 : Step  Time=Tfault+Ts_Power  SampleTime=Ts_Power
  BL11 : Step  Time=Tfault  SampleTime=Ts_Power
  BL2 : Step  Time=Tbrk2_On  SampleTime=Ts_Power
  BL3 : Step  Time=Ton_Converter2  SampleTime=Ts_Power
  BL4 : Step  Time=Ton_VDCreg  SampleTime=Ts
  BL5 : Step  Time=Tdeblock  Before=1  After=0  SampleTime=Ts_Power
  BL6 : Step  Time=Ton_PQreg  SampleTime=Ts
  BL8 : Step  Time=Tfault + 1.95*(1/Fnom)  Before=1  After=0  SampleTime=Ts_Power
  BL9 : Step  Time=Tfault + 2*(1/Fnom)  Before=1  After=0  SampleTime=Ts_Power
  Logical Operator : Logic  AllPortsSameDT=off  OutDataTypeStr=boolean
  Logical Operator1 : Logic  Operator=OR  AllPortsSameDT=off  OutDataTypeStr=float('double')
  Logical Operator2 : Logic  AllPortsSameDT=off  OutDataTypeStr=boolean
  Pref : simulink/Sources/Ramp  slope=Slope_Pref  start=Tramping_Pref  InitialOutput=0
  Qref : simulink/Sources/Ramp  slope=Slope_Qref  start=Tramping_Qref  InitialOutput=0
  Rate Transition3 : RateTransition  OutPortSampleTime=Ts_Control
  Rate Transition4 : RateTransition  OutPortSampleTime=Ts_Control
  Rate Transition5 : RateTransition  OutPortSampleTime=Ts_Control
  Saturation : Saturate  UpperLimit=1  LowerLimit=-1
  Saturation1 : Saturate  UpperLimit=Limits_Qreg(1)  LowerLimit=Limits_Qreg(2)
  Saturation2 : Saturate  UpperLimit=Vnom_dc  LowerLimit=eps
  "Vdc_ref " : simulink/Sources/Ramp  slope=Slope_Vdc_ref  start=Tramping_Vdc_ref  InitialOutput=Vnom_sec*1.37
  tag scope: Blk=global, Brk1_On=global, Brk2_On=global, Converter2_On=global, Fault_On=global, PQreg_On=global, Pref=global, Qref=global, VDCreg_On=global, Vdc_ref=global
  wires:
  Saturation2/1 -> Rate Transition5/1
  Saturation1/1 -> Rate Transition4/1
  Pref/1 -> Saturation/1
  Qref/1 -> Saturation1/1
  Saturation/1 -> Rate Transition3/1
  Rate Transition3/1 -> [Pref]
  Rate Transition4/1 -> [Qref]
  Rate Transition5/1 -> [Vdc_ref]
  BL4/1 -> [VDCreg_On]
  BL6/1 -> [PQreg_On]
  "Vdc_ref "/1 -> Saturation2/1
  BL2/1 -> [Brk2_On]
  BL8/1 -> Logical Operator/2
  Logical Operator/1 -> [Brk1_On]
  BL1/1 -> Logical Operator/1
  BL9/1 -> Logical Operator2/2
  BL3/1 -> Logical Operator2/1
  Logical Operator2/1 -> [Converter2_On]
  Logical Operator1/1 -> [Blk]
  BL5/1 -> Logical Operator1/1
  BL10/1 -> Logical Operator1/2
  BL11/1 -> [Fault_On]

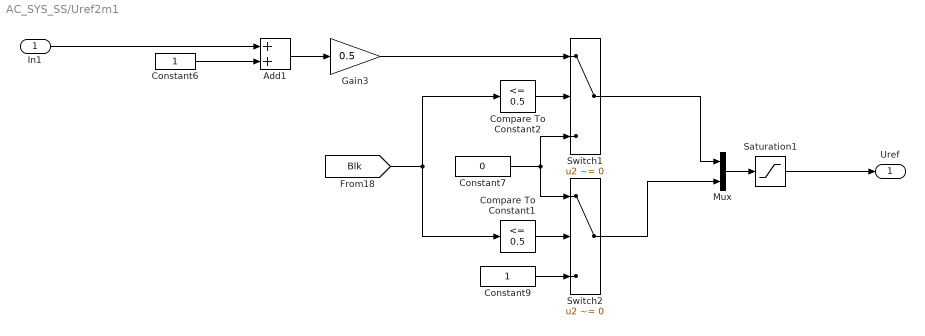
== system AC_SYS_SS/Uref2m1 ==
  In1 : Inport
  Add1 : Sum
  Compare To Constant1 : simulink/Logic and Bit Operations/Compare To Constant  relop=<=  const=0.5  OutDataTypeStr=boolean
  Compare To Constant2 : simulink/Logic and Bit Operations/Compare To Constant  relop=<=  const=0.5  OutDataTypeStr=boolean
  Constant6 : Constant
  Constant7 : Constant  Value=0
  Constant9 : Constant
  Gain3 : Gain  Gain=0.5
  Mux : Mux  Inputs=2
  Saturation1 : Saturate  UpperLimit=1  LowerLimit=0
  Switch1 : Switch  Criteria=u2 ~= 0  SaturateOnIntegerOverflow=off  InputSameDT=off
  Switch2 : Switch  Criteria=u2 ~= 0  SaturateOnIntegerOverflow=off  InputSameDT=off
  Uref : Outport
  wires:
  Switch1/1 -> Mux/1
  [Blk] -> Compare To Constant1/1, Compare To Constant2/1
  Add1/1 -> Gain3/1
  Gain3/1 -> Switch1/1
  Constant7/1 -> Switch1/3, Switch2/1
  Compare To Constant1/1 -> Switch2/2
  Constant6/1 -> Add1/2
  Mux/1 -> Saturation1/1
  Constant9/1 -> Switch2/3
  Compare To Constant2/1 -> Switch1/2
  Switch2/1 -> Mux/2
  In1/1 -> Add1/1
  Saturation1/1 -> Uref/1

== system AC_SYS_SS/Voltage source ==
  In1 : Inport
  Demux9 : Demux  Outputs=3
  Ground : spsGroundLib/Ground  LConnTagsString=a
  VSRC_a : spsControlledVoltageSourceLib/Controlled Voltage Source  Initialize=on  Source_Type=AC  Amplitude=0  Phase=0  Frequency=0  Measurements=None
  VSRC_b : spsControlledVoltageSourceLib/Controlled Voltage Source  Initialize=on  Source_Type=AC  Amplitude=0  Phase=0  Frequency=0  Measurements=None
  VSRC_c : spsControlledVoltageSourceLib/Controlled Voltage Source  Initialize=on  Source_Type=AC  Amplitude=0  Phase=0  Frequency=0  Measurements=None
  a : PMIOPort  Side=Right
  b : PMIOPort  Port=2  Side=Right
  c : PMIOPort  Port=3  Side=Right
  wires:
  In1/1 -> Demux9/1
  Demux9/1 -> VSRC_a/1
  Demux9/2 -> VSRC_b/1
  Demux9/3 -> VSRC_c/1
  connections:
  Ground/LConn1 -- VSRC_b/LConn1 -- VSRC_a/LConn1 -- VSRC_c/LConn1
  VSRC_c/RConn1 -- c/RConn1
  VSRC_b/RConn1 -- b/RConn1
  VSRC_a/RConn1 -- a/RConn1

== system AC_SYS_SS/param ==

== system AC_SYS_SS/BRK_CTRL/MUX2 ==
  In1 : Inport
  In2 : Inport  Port=2
  Demux4 : Demux  Outputs=3
  Demux5 : Demux  Outputs=3
  Mux13 : Mux  Inputs=2
  Mux14 : Mux  Inputs=2
  Mux15 : Mux  Inputs=3
  Mux8 : Mux  Inputs=2
  Sum1 : Sum  Inputs=1  InputSameDT=on  SaturateOnIntegerOverflow=on  OutDataTypeStr=Inherit: Same as first input
  Sum4 : Sum  Inputs=1  InputSameDT=on  SaturateOnIntegerOverflow=on  OutDataTypeStr=Inherit: Same as first input
  Sum5 : Sum  Inputs=1  InputSameDT=on  SaturateOnIntegerOverflow=on  OutDataTypeStr=Inherit: Same as first input
  Out1 : Outport
  wires:
  Demux5/3 -> Mux14/2
  In1/1 -> Demux4/1
  Demux4/1 -> Mux8/1
  Demux5/1 -> Mux8/2
  In2/1 -> Demux5/1
  Sum1/1 -> Mux15/1
  Demux5/2 -> Mux13/2
  Mux14/1 -> Sum5/1
  Mux8/1 -> Sum1/1
  Demux4/2 -> Mux13/1
  Mux13/1 -> Sum4/1
  Sum5/1 -> Mux15/3
  Sum4/1 -> Mux15/2
  Demux4/3 -> Mux14/1
  Mux15/1 -> Out1/1

== system AC_SYS_SS/BRK_CTRL1/MUX2 ==
  In1 : Inport
  In2 : Inport  Port=2
  Demux4 : Demux  Outputs=3
  Demux5 : Demux  Outputs=3
  Mux13 : Mux  Inputs=2
  Mux14 : Mux  Inputs=2
  Mux15 : Mux  Inputs=3
  Mux8 : Mux  Inputs=2
  Sum1 : Sum  Inputs=1  InputSameDT=on  SaturateOnIntegerOverflow=on  OutDataTypeStr=Inherit: Same as first input
  Sum4 : Sum  Inputs=1  InputSameDT=on  SaturateOnIntegerOverflow=on  OutDataTypeStr=Inherit: Same as first input
  Sum5 : Sum  Inputs=1  InputSameDT=on  SaturateOnIntegerOverflow=on  OutDataTypeStr=Inherit: Same as first input
  Out1 : Outport
  wires:
  Demux5/3 -> Mux14/2
  In1/1 -> Demux4/1
  Demux4/1 -> Mux8/1
  Demux5/1 -> Mux8/2
  In2/1 -> Demux5/1
  Sum1/1 -> Mux15/1
  Demux5/2 -> Mux13/2
  Mux14/1 -> Sum5/1
  Mux8/1 -> Sum1/1
  Demux4/2 -> Mux13/1
  Mux13/1 -> Sum4/1
  Sum5/1 -> Mux15/3
  Sum4/1 -> Mux15/2
  Demux4/3 -> Mux14/1
  Mux15/1 -> Out1/1
